simulink model "if_and_looping"  (R2021a)
settings: Solver=FixedStepDiscrete  StartTime=0.0  StopTime=10.0  RelTol=1e-3  EnableMultiTasking=on
settings Model: Creator=Mahmoud Sofar  LastModifiedBy=Mahmoud Sofar
settings DataIOCC: ReturnWorkspaceOutputs=off
settings OptimizationCC: DefaultParameterBehavior=Inlined  InlineInvariantSignals=on  EnableMemcpy=off  LifeSpan=1  EfficientTunableParamExpr=on
settings DebuggingCC: UnderspecifiedInitializationDetection=Classic  MergeDetectMultiDrivingBlocksExec=none  SFMachineParentedDataDiag=warning  ArithmeticOperatorsInVariantConditions=warning
settings ModelReferenceCC: PropagateSignalLabelsOutOfModel=off
settings SFSimCC: MATLABDynamicMemAlloc=off  CustomCodeUndefinedFunction=UseInterfaceOnly
settings RTWCC: SystemTargetFile=ert.tlc  GenCodeOnly=on  TemplateMakefile=ert_default_tmf  GenerateReport=on  IncludeHyperlinkInReport=on  LaunchReport=on  GenerateTraceInfo=on  GenerateTraceReport=on  GenerateTraceReportSl=on  GenerateTraceReportSf=on  GenerateTraceReportEml=on
settings CodeAppCC: ForceParamTrailComments=on  IgnoreCustomStorageClasses=off  OperatorAnnotations=on  SimulinkDataObjDesc=on  SFDataObjDesc=on  MATLABFcnDesc=on  InsertBlockDesc=on  StateflowObjectComments=on  MATLABSourceComments=on
settings ERTTargetCC: MultiwordLength=2048  GenerateSampleERTMain=on  InlinedParameterPlacement=NonHierarchical  ERTCustomFileTemplate=example_file_process.tlc

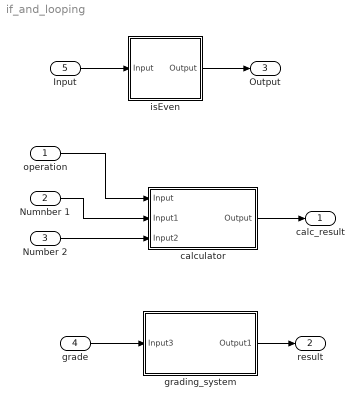
== system if_and_looping ==
  operation : Inport
  Numnber 1 : Inport  Port=2
  Number 2 : Inport  Port=3
  grade : Inport  Port=4
  Input : Inport  Port=5  OutDataTypeStr=uint32
  calculator : Subsystem  TreatAsAtomicUnit=on
      settings: RTWFcnNameOpts=Use subsystem name  RTWFileNameOpts=Use function name
  grading_system : Subsystem  TreatAsAtomicUnit=on
      settings: RTWFcnNameOpts=Use subsystem name  RTWFileNameOpts=Use subsystem name
  isEven : Subsystem  TreatAsAtomicUnit=on
      settings: RTWFcnNameOpts=Use subsystem name  RTWFileNameOpts=Use subsystem name
  calc_result : Outport
  result : Outport  Port=2  OutDataTypeStr=string
  Output : Outport  Port=3
  wires:
  operation/1 -> calculator/1(Input)
  Numnber 1/1 -> calculator/2(Input1)
  Number 2/1 -> calculator/3(Input2)
  calculator/1(Output) -> calc_result/1
  grade/1 -> grading_system/1(Input3)
  grading_system/1(Output1) -> result/1
  Input/1 -> isEven/1(Input)
  isEven/1(Output) -> Output/1

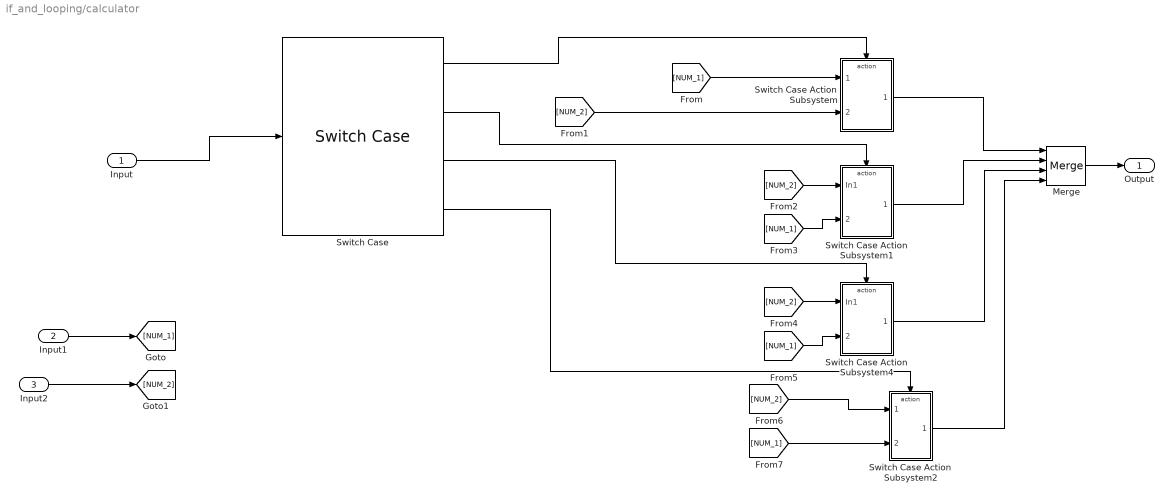
== system if_and_looping/calculator ==
  Input : Inport  OutDataTypeStr=uint32
  Input1 : Inport  Port=2
  Input2 : Inport  Port=3
  Merge : Merge  Inputs=4
  Switch Case : SwitchCase  CaseConditions={0,1,2,3}  ShowDefaultCase=off
  Switch Case Action Subsystem : Subsystem  TreatAsAtomicUnit=on
  Switch Case Action Subsystem1 : Subsystem  TreatAsAtomicUnit=on
  Switch Case Action Subsystem2 : Subsystem  TreatAsAtomicUnit=on
  Switch Case Action Subsystem4 : Subsystem  TreatAsAtomicUnit=on
  Output : Outport
  wires:
  Switch Case/4 -> Switch Case Action Subsystem2/Action
  [NUM_1] -> Switch Case Action Subsystem1/2(Input)
  Switch Case/3 -> Switch Case Action Subsystem4/Action
  Switch Case/1 -> Switch Case Action Subsystem/Action
  Merge/1 -> Output/1
  Input1/1 -> [NUM_1]
  Switch Case Action Subsystem/1(Out1) -> Merge/1
  Switch Case Action Subsystem2/1(Out1) -> Merge/4
  [NUM_1] -> Switch Case Action Subsystem/1(Input1)
  Switch Case/2 -> Switch Case Action Subsystem1/Action
  Input2/1 -> [NUM_2]
  [NUM_2] -> Switch Case Action Subsystem2/1(In1)
  [NUM_1] -> Switch Case Action Subsystem4/2(Input)
  [NUM_2] -> Switch Case Action Subsystem4/1(In1)
  [NUM_2] -> Switch Case Action Subsystem/2(Input)
  Input/1 -> Switch Case/1
  [NUM_1] -> Switch Case Action Subsystem2/2(Input)
  Switch Case Action Subsystem4/1(Out1) -> Merge/3
  Switch Case Action Subsystem1/1(Out1) -> Merge/2
  [NUM_2] -> Switch Case Action Subsystem1/1(In1)

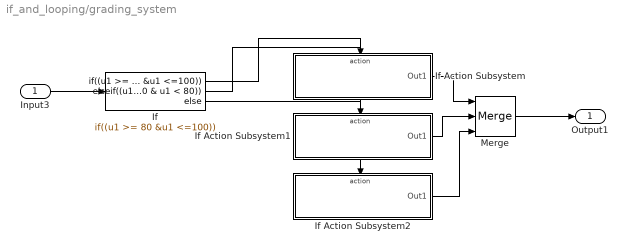
== system if_and_looping/grading_system ==
  Input3 : Inport
  If : If  IfExpression=(u1 >= 80 &u1 <=100)  ElseIfExpressions=(u1 > 50 & u1 < 80)
  If Action Subsystem : Subsystem  TreatAsAtomicUnit=on
  If Action Subsystem1 : Subsystem  TreatAsAtomicUnit=on
  If Action Subsystem2 : Subsystem  TreatAsAtomicUnit=on
  Merge : Merge  Inputs=3
  Output1 : Outport  OutDataTypeStr=string
  wires:
  If Action Subsystem/1(Out1) -> Merge/1
  Merge/1 -> Output1/1
  If Action Subsystem1/1(Out1) -> Merge/2
  If/3 -> If Action Subsystem2/Action
  If/2 -> If Action Subsystem1/Action
  If Action Subsystem2/1(Out1) -> Merge/3
  Input3/1 -> If/1
  If/1 -> If Action Subsystem/Action

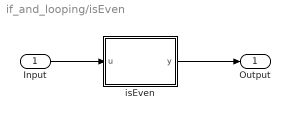
== system if_and_looping/isEven ==
  Input : Inport  OutDataTypeStr=uint32
  isEven : MATLAB Function  TreatAsAtomicUnit=on
  Output : Outport
  wires:
  Input/1 -> isEven/1(u)
  isEven/1(y) -> Output/1

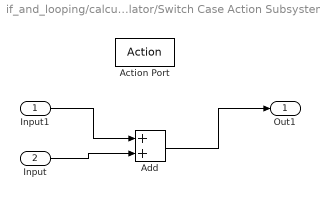
== system if_and_looping/calculator/Switch Case Action Subsystem ==
  Input1 : Inport
  Input : Inport  Port=2
  Action Port : ActionPort  ActionPortLabel=case [ 0 ]:
  Add : Sum
  Out1 : Outport
  wires:
  Input1/1 -> Add/1
  Input/1 -> Add/2
  Add/1 -> Out1/1

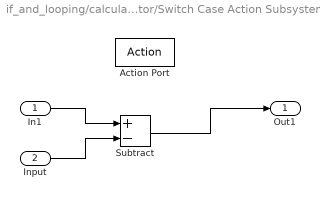
== system if_and_looping/calculator/Switch Case Action Subsystem1 ==
  In1 : Inport
  Input : Inport  Port=2
  Action Port : ActionPort  ActionPortLabel=case [ 1 ]:
  Subtract : Sum  Inputs=+-
  Out1 : Outport
  wires:
  In1/1 -> Subtract/1
  Input/1 -> Subtract/2
  Subtract/1 -> Out1/1

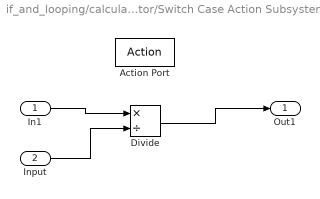
== system if_and_looping/calculator/Switch Case Action Subsystem2 ==
  In1 : Inport
  Input : Inport  Port=2
  Action Port : ActionPort  ActionPortLabel=case [ 3 ]:
  Divide : Product  Inputs=*/
  Out1 : Outport
  wires:
  In1/1 -> Divide/1
  Input/1 -> Divide/2
  Divide/1 -> Out1/1

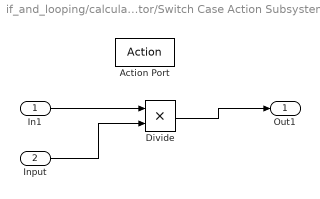
== system if_and_looping/calculator/Switch Case Action Subsystem4 ==
  In1 : Inport
  Input : Inport  Port=2
  Action Port : ActionPort  ActionPortLabel=case [ 2 ]:
  Divide : Product  Inputs=**
  Out1 : Outport
  wires:
  In1/1 -> Divide/1
  Input/1 -> Divide/2
  Divide/1 -> Out1/1

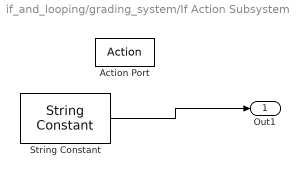
== system if_and_looping/grading_system/If Action Subsystem ==
  Action Port : ActionPort  ActionPortLabel=if((u1 >= 80 &u1 <=100))
  String Constant : StringConstant  String="\"Excellent\""
  Out1 : Outport  OutDataTypeStr=string
  wires:
  String Constant/1 -> Out1/1

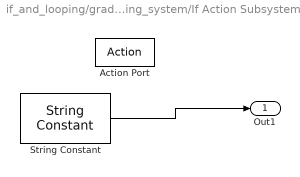
== system if_and_looping/grading_system/If Action Subsystem1 ==
  Action Port : ActionPort  ActionPortLabel=elseif((u1 > 50 & u1 < 80))
  String Constant : StringConstant  String="\"Pass\""
  Out1 : Outport  OutDataTypeStr=string
  wires:
  String Constant/1 -> Out1/1

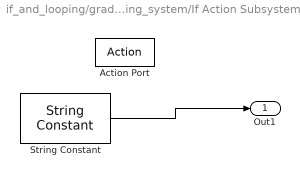
== system if_and_looping/grading_system/If Action Subsystem2 ==
  Action Port : ActionPort  ActionPortLabel=else
  String Constant : StringConstant  String="\"Fail\""
  Out1 : Outport  OutDataTypeStr=string
  wires:
  String Constant/1 -> Out1/1

== matlab function if_and_looping/isEven/isEven ==
  data: u input; y output
function y = fcn(u)
if mod(u, 2) == 0
    y = 1;
else 
    y = 0;
end   
end
